simulink model "gauss_mf1"  (R2016a)
settings: Solver=VariableStepAuto  StartTime=0.0  StopTime=10.0  RelTol=1e-3
undefined symbols (not defined in the file): fi_1_mu, fi_1_sigma
settings Model: Creator=Руслан  LastModifiedBy=Руслан

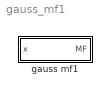
== system gauss_mf1 ==
  gauss mf1 : Subsystem  mask{sigma=fi_1_sigma, mu=fi_1_mu}
      mask prompts: sigma "Variance sigma:"; mu "Mean c:"

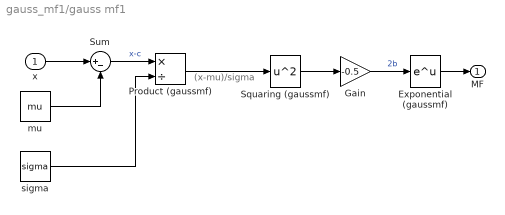
== system gauss_mf1/gauss mf1 ==
  note: (x-mu)/sigma
  x : Inport
  Exponential (gaussmf) : Math  SaturateOnIntegerOverflow=on
  Gain : Gain  Gain=-0.5  SaturateOnIntegerOverflow=on  OutDataTypeStr=Inherit: Same as input  ParamDataTypeStr=Inherit: Same as input
  Product (gaussmf) : Product  Inputs=*/  SaturateOnIntegerOverflow=on  InputSameDT=on  OutDataTypeStr=Inherit: Same as first input
  Squaring (gaussmf) : Math  Operator=square  SaturateOnIntegerOverflow=on
  Sum : Sum  Inputs=|+-  SaturateOnIntegerOverflow=on  InputSameDT=on  OutDataTypeStr=Inherit: Same as first input
  mu : Constant  Value=mu
  sigma : Constant  Value=sigma
  MF : Outport
  wires:
  Product (gaussmf)/1 -> Squaring (gaussmf)/1
  Gain/1 -> Exponential (gaussmf)/1  "2b"
  Squaring (gaussmf)/1 -> Gain/1
  Exponential (gaussmf)/1 -> MF/1
  sigma/1 -> Product (gaussmf)/2
  Sum/1 -> Product (gaussmf)/1  "x-c"
  mu/1 -> Sum/2
  x/1 -> Sum/1
